simulink model "eg_2_01_02_R2023a"  (R2023a)
settings: Solver=ode4  StartTime=0.0  StopTime=10  FixedStep=0.001  RelTol=1e-3  EnableMultiTasking=on
values from neighbouring files (symbols this model uses):
  c = 0.695    [aaa.m]    (also in eg_2_01_02.m; eg_2_03.m = [ diff( y,x1) diff( y,x2) ]; eg_2_04.m = subs(c,{M1,M2,k,mu},{0.5,1,2,1}); eg_2_05.m = [ diff( y,x1) diff( y,x2) ])
  g = 9.81    [aaa.m]    (also in eg_2_01_02.m)
  J = 0.0712    [aaa.m]    (also in eg_2_01_02.m)
  l = 0.204    [aaa.m]    (also in eg_2_01_02.m)
  M = 0.390    (= 0.39)    [aaa.m]    (also in eg_2_01_02.m)
settings Model: Creator=kawata  LastModifiedBy=kawata
settings SolverCC: AlgebraicLoopSolver=TrustRegion
settings DataIOCC: LimitDataPoints=on  SaveFormat=Array  SignalLoggingSaveFormat=ModelDataLogs  ReturnWorkspaceOutputs=off  SignalLoggingName=sigsOut
settings OptimizationCC: ExpressionDepthLimit=2147483647  LifeSpan=inf
settings DebuggingCC: SaveWithParameterizedLinksMsg=none  UnderspecifiedInitializationDetection=Classic  MergeDetectMultiDrivingBlocksExec=none  SignalResolutionControl=TryResolveAllWithWarning  MultiTaskDSMMsg=warning  MultiTaskCondExecSysMsg=none  FcnCallInpInsideContextMsg=warning  UnconnectedInputMsg=warning  UnconnectedOutputMsg=warning  UnconnectedLineMsg=warning  StateNameClashWarn=warning  SFUnexpectedBacktrackingDiag=warning  SFNoUnconditionalDefaultTransitionDiag=warning  SFExecutionAtInitializationDiag=none  ArithmeticOperatorsInVariantConditions=warning
settings HardwareCC: ProdBitPerPointer=32  ProdBitPerSizeT=32  ProdBitPerPtrDiffT=32  ProdLargestAtomicFloat=None  ProdIntDivRoundTo=Undefined  ProdEndianess=Unspecified  ProdWordSize=32  ProdHWDeviceType=32-bit Generic  TargetUnknown=on
settings ModelReferenceCC: EnableRefExpFcnMdlSchedulingChecks=on  PropagateSignalLabelsOutOfModel=off
settings SFSimCC: SimUseLocalCustomCode=off  CustomCodeUndefinedFunction=UseInterfaceOnly
settings RTWCC: RTWUseLocalCustomCode=off
settings CodeAppCC: StateflowObjectComments=on
settings GRTTargetCC: TargetLangStandard=C89/C90 (ANSI)  CombineOutputUpdateFcns=off  GRTInterface=on
settings ConfigComp: CovMetricSettings=dw  CovSaveCumulativeToWorkspaceVar=on  CovSaveSingleToWorkspaceVar=on  CovExternalEMLEnable=off

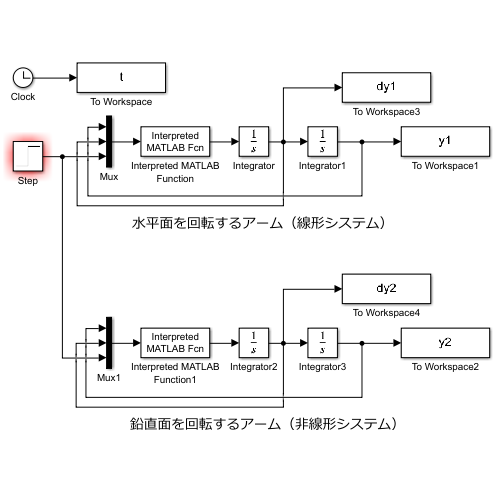
[thumbnail: Simulink's stored preview of the top-level diagram]
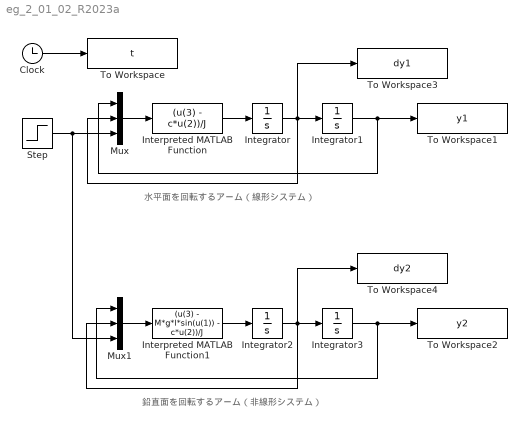
== system eg_2_01_02_R2023a ==
  note: 鉛直面を回転するアーム（非線形システム）
  note: 水平面を回転するアーム（線形システム）
  Clock : Clock
  Integrator{,1..3} (4 alike) : Integrator
  Interpreted MATLAB Function : MATLABFcn  MATLABFcn=(u(3) - c*u(2))/J
  Interpreted MATLAB Function1 : MATLABFcn  MATLABFcn=(u(3) - M*g*l*sin(u(1)) - c*u(2))/J
  Mux : Mux  Inputs=3
  Mux1 : Mux  Inputs=3
  Step : Step  Time=0  After=u  SampleTime=0
  To Workspace : ToWorkspace  VariableName=t  SampleTime=-1
  To Workspace1 : ToWorkspace  VariableName=y1  SampleTime=-1
  To Workspace2 : ToWorkspace  VariableName=y2  SampleTime=-1
  To Workspace3 : ToWorkspace  VariableName=dy1  SampleTime=-1
  To Workspace4 : ToWorkspace  VariableName=dy2  SampleTime=-1
  wires:
  Interpreted MATLAB Function/1 -> Integrator/1
  Integrator/1 -> To Workspace3/1, Integrator1/1, Mux/2
  Mux/1 -> Interpreted MATLAB Function/1
  Step/1 -> Mux/3, Mux1/3
  Integrator1/1 -> To Workspace1/1, Mux/1
  Clock/1 -> To Workspace/1
  Interpreted MATLAB Function1/1 -> Integrator2/1
  Integrator2/1 -> To Workspace4/1, Integrator3/1, Mux1/2
  Mux1/1 -> Interpreted MATLAB Function1/1
  Integrator3/1 -> To Workspace2/1, Mux1/1
